simulink model "Junctions2"  (Simulink 5.0)
settings: Solver=ode45  StartTime=0.0  StopTime=10.0  RelTol=1e-3
settings Model: Creator=scaife  LastModifiedBy=scaife  ExtModeAutoUpdateStatusClock=off

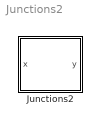
== system Junctions2 ==
  Junctions2 : Stateflow chart

== stateflow chart Junctions2 ==
  state A
  state B
  state C
  state D
  (default) -> A
  A -> (junction 7) : [x>0]{y++}
  (junction 7) -> B : [x<2]{y+=10}
  (junction 7) -> (junction 8) : [x>=2]{y+=100}
  (junction 8) -> C : [x<4]{y+=1000}
  (junction 8) -> D : [x>=4]
      | {y+=10000}
  B -> C : [x==0]
  C -> D : [x==0]
  D -> A : [x==0]
  data: x input int32; y output int32 =11111
